simulink model "Hybrid_vehicle_MIL"  (R2020b)
settings: configuration reference "gen_config" (kept outside this file)
settings Model: DataDictionary=Hybrid_vehicle.sldd  SimulationMode=accelerator  Creator=Georg  LastModifiedBy=jy
settings ConfigSetRef: SourceName=gen_config

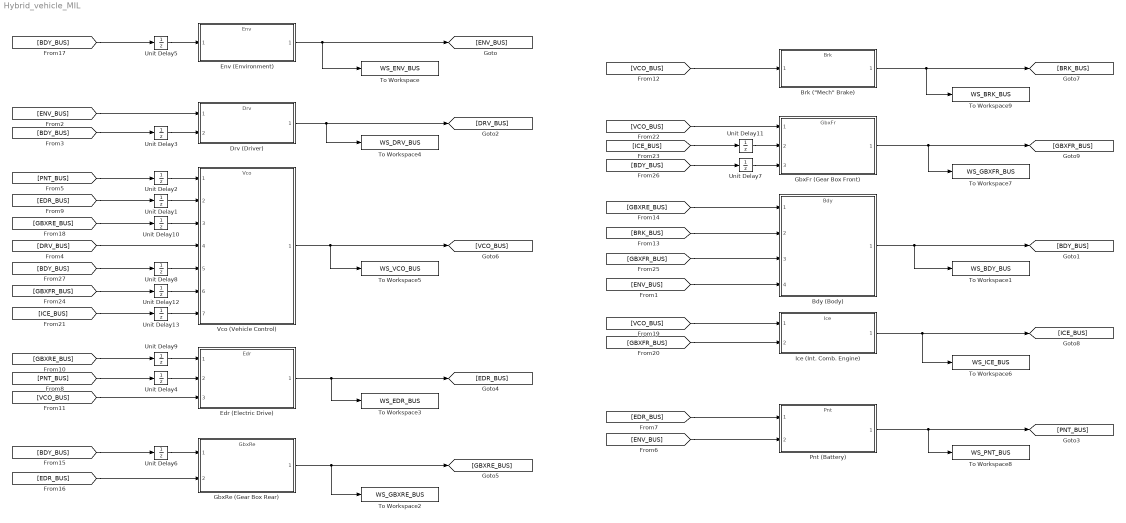
== system Hybrid_vehicle_MIL ==
  Bdy (Body) : ModelReference  ModelNameDialog=Bdy  SimulationMode=Normal  ModelReferenceVersion=2.38
  "Brk (\"Mech\" Brake)" : ModelReference  ModelNameDialog=Brk  SimulationMode=Normal  ModelReferenceVersion=2.30
  Drv (Driver) : ModelReference  ModelNameDialog=Drv  SimulationMode=Normal  ModelReferenceVersion=2.29
  Edr (Electric Drive) : ModelReference  ModelNameDialog=Edr  SimulationMode=Normal  ModelReferenceVersion=2.38
  Env (Environment) : ModelReference  ModelNameDialog=Env  SimulationMode=Normal  ModelReferenceVersion=2.22
  GbxFr (Gear Box Front) : ModelReference  ModelNameDialog=GbxFr  SimulationMode=Normal  ModelReferenceVersion=2.27
  GbxRe (Gear Box Rear) : ModelReference  ModelNameDialog=GbxRe  SimulationMode=Normal  ModelReferenceVersion=2.25
  Ice (Int. Comb. Engine) : ModelReference  ModelNameDialog=Ice  SimulationMode=Normal  ModelReferenceVersion=2.29
  Pnt (Battery) : ModelReference  ModelNameDialog=Pnt  SimulationMode=Normal  ModelReferenceVersion=2.35
  To Workspace : ToWorkspace  VariableName=WS_ENV_BUS  SaveFormat=Timeseries  SampleTime=-1
  To Workspace1 : ToWorkspace  VariableName=WS_BDY_BUS  SaveFormat=Timeseries  SampleTime=-1
  To Workspace2 : ToWorkspace  VariableName=WS_GBXRE_BUS  SaveFormat=Timeseries  SampleTime=-1
  To Workspace3 : ToWorkspace  VariableName=WS_EDR_BUS  SaveFormat=Timeseries  SampleTime=-1
  To Workspace4 : ToWorkspace  VariableName=WS_DRV_BUS  SaveFormat=Timeseries  SampleTime=-1
  To Workspace5 : ToWorkspace  VariableName=WS_VCO_BUS  SaveFormat=Timeseries  SampleTime=-1
  To Workspace6 : ToWorkspace  VariableName=WS_ICE_BUS  SaveFormat=Timeseries  SampleTime=-1
  To Workspace7 : ToWorkspace  VariableName=WS_GBXFR_BUS  SaveFormat=Timeseries  SampleTime=-1
  To Workspace8 : ToWorkspace  VariableName=WS_PNT_BUS  SaveFormat=Timeseries  SampleTime=-1
  To Workspace9 : ToWorkspace  VariableName=WS_BRK_BUS  SaveFormat=Timeseries  SampleTime=-1
  Unit Delay{1..13} (13 alike) : UnitDelay  SampleTime=-1  HasFrameUpgradeWarning=on
  Vco (Vehicle Control) : ModelReference  ModelNameDialog=Vco  SimulationMode=Normal  ModelReferenceVersion=2.42
  wires:
  [ENV_BUS] -> Bdy (Body)/4
  Vco (Vehicle Control)/1 -> [VCO_BUS], To Workspace5/1
  [PNT_BUS] -> Unit Delay2/1
  [ICE_BUS] -> Unit Delay13/1
  [GBXRE_BUS] -> Bdy (Body)/1
  Unit Delay1/1 -> Vco (Vehicle Control)/2
  [EDR_BUS] -> Unit Delay1/1
  Unit Delay2/1 -> Vco (Vehicle Control)/1
  [ENV_BUS] -> Drv (Driver)/1
  [BDY_BUS] -> Unit Delay3/1
  [DRV_BUS] -> Vco (Vehicle Control)/4
  Pnt (Battery)/1 -> [PNT_BUS], To Workspace8/1
  [ENV_BUS] -> Pnt (Battery)/2
  [EDR_BUS] -> Pnt (Battery)/1
  Unit Delay4/1 -> Edr (Electric Drive)/2
  [PNT_BUS] -> Unit Delay4/1
  [GBXRE_BUS] -> Unit Delay9/1
  [VCO_BUS] -> Edr (Electric Drive)/3
  [BRK_BUS] -> Bdy (Body)/2
  [BDY_BUS] -> Unit Delay6/1
  [EDR_BUS] -> GbxRe (Gear Box Rear)/2
  [GBXRE_BUS] -> Unit Delay10/1
  [VCO_BUS] -> Ice (Int. Comb. Engine)/1
  [GBXFR_BUS] -> Ice (Int. Comb. Engine)/2
  GbxRe (Gear Box Rear)/1 -> [GBXRE_BUS], To Workspace2/1
  Edr (Electric Drive)/1 -> [EDR_BUS], To Workspace3/1
  [VCO_BUS] -> GbxFr (Gear Box Front)/1
  [ICE_BUS] -> Unit Delay11/1
  [GBXFR_BUS] -> Unit Delay12/1
  [GBXFR_BUS] -> Bdy (Body)/3
  [BDY_BUS] -> Unit Delay7/1
  [BDY_BUS] -> Unit Delay8/1
  Env (Environment)/1 -> [ENV_BUS], To Workspace/1
  Drv (Driver)/1 -> [DRV_BUS], To Workspace4/1
  GbxFr (Gear Box Front)/1 -> To Workspace7/1, [GBXFR_BUS]
  Ice (Int. Comb. Engine)/1 -> To Workspace6/1, [ICE_BUS]
  Bdy (Body)/1 -> [BDY_BUS], To Workspace1/1
  [BDY_BUS] -> Unit Delay5/1
  Unit Delay3/1 -> Drv (Driver)/2
  Unit Delay5/1 -> Env (Environment)/1
  Unit Delay6/1 -> GbxRe (Gear Box Rear)/1
  Unit Delay7/1 -> GbxFr (Gear Box Front)/3
  Unit Delay8/1 -> Vco (Vehicle Control)/5
  Unit Delay9/1 -> Edr (Electric Drive)/1
  Unit Delay10/1 -> Vco (Vehicle Control)/3
  Unit Delay11/1 -> GbxFr (Gear Box Front)/2
  Unit Delay12/1 -> Vco (Vehicle Control)/6
  Unit Delay13/1 -> Vco (Vehicle Control)/7
  "Brk (\"Mech\" Brake)"/1 -> [BRK_BUS], To Workspace9/1
  [VCO_BUS] -> "Brk (\"Mech\" Brake)"/1
